simulink model "Lab_6b"  (R2014a)
settings: Solver=ode23t  StartTime=0.0  StopTime=20  RelTol=1e-3
settings Model: Creator=cloughj  LastModifiedBy=cloughj
settings SolverCC: ZeroCrossAlgorithm=Adaptive

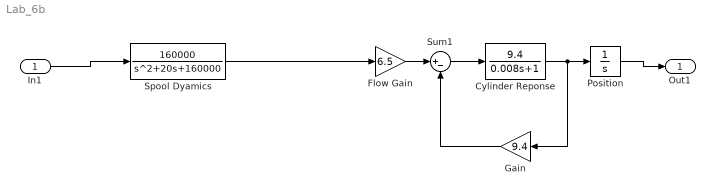
== system Lab_6b ==
  In1 : Inport
  Cylinder Reponse : TransferFcn  Numerator=[9.4]  Denominator="[0.008  1]"
  Flow Gain : Gain  Gain=6.5
  Gain : Gain  Gain=9.4
  Position : Integrator
  Spool Dyamics : TransferFcn  Numerator=[160000]  Denominator=[1 20 160000]
  Sum1 : Sum  Inputs=|+-
  Out1 : Outport
  wires:
  Flow Gain/1 -> Sum1/1
  Sum1/1 -> Cylinder Reponse/1
  Cylinder Reponse/1 -> Gain/1, Position/1
  Gain/1 -> Sum1/2
  In1/1 -> Spool Dyamics/1
  Spool Dyamics/1 -> Flow Gain/1
  Position/1 -> Out1/1
